simulink model "GearedShaft_Q1_1"  (R2026a)
settings: Solver=ode4  StopTime=1  FixedStep=1e-5

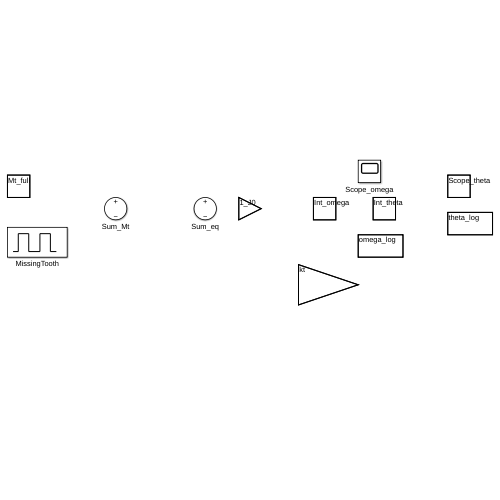
[thumbnail: Simulink's stored preview of the top-level diagram]
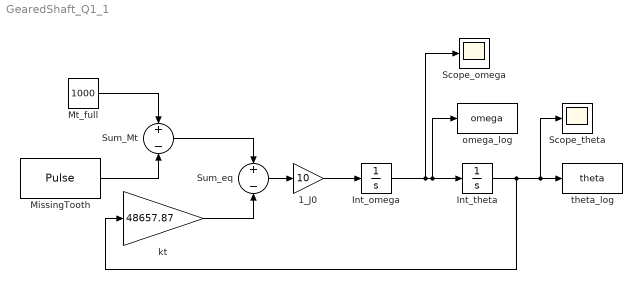
== system GearedShaft_Q1_1 ==
  1_J0 : Gain  Gain=10
  Int_omega : Integrator
  Int_theta : Integrator  InitialCondition=0.02055
  MissingTooth : DiscretePulseGenerator  PulseType=Time based  Amplitude=1000  Period=0.06  PulseWidth=6.25
  Mt_full : Constant  Value=1000
  Scope_omega : Scope
  Scope_theta : Scope
  Sum_Mt : Sum  Inputs=+-
  Sum_eq : Sum  Inputs=+-
  kt : Gain  Gain=48657.87
  omega_log : ToWorkspace  VariableName=omega  SaveFormat=Timeseries  SampleTime=-1
  theta_log : ToWorkspace  VariableName=theta  SaveFormat=Timeseries  SampleTime=-1
  wires:
  Int_theta/1 -> theta_log/1, Scope_theta/1, kt/1
  Int_omega/1 -> omega_log/1, Int_theta/1, Scope_omega/1
  Sum_eq/1 -> 1_J0/1
  kt/1 -> Sum_eq/2
  Sum_Mt/1 -> Sum_eq/1
  1_J0/1 -> Int_omega/1
  MissingTooth/1 -> Sum_Mt/2
  Mt_full/1 -> Sum_Mt/1
